simulink model "problem3_ccmodel"  (R2020a)
settings: Solver=VariableStepAuto  StartTime=0.0  StopTime=10.0  RelTol=1e-3
model workspace (MAT data in the model file):
  b = 50
  kd = 50
  ki = 300
  kp = 350
  m = 1000
  u = 500
settings Model: DataDictionary=poblem3_ccmodel.sldd  Creator=HP  LastModifiedBy=HP

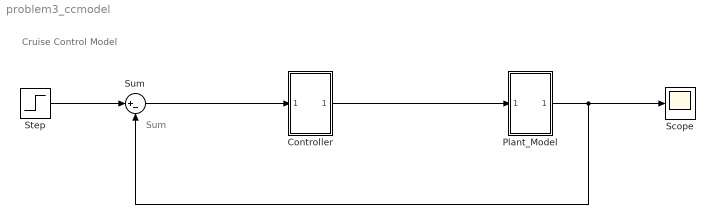
== system problem3_ccmodel ==
  note: Cruise Control Model
  note: Sum
  Controller : Subsystem  TreatAsAtomicUnit=on
  Plant_Model : Subsystem
  Scope : Scope
  Step : Step  Time=0  After=u  SampleTime=0
  Sum : Sum  Inputs=|+-
  wires:
  Step/1 -> Sum/1
  Plant_Model/1(Out1) -> Scope/1, Sum/2
  Sum/1 -> Controller/1(In1)
  Controller/1(Out1) -> Plant_Model/1(In1)

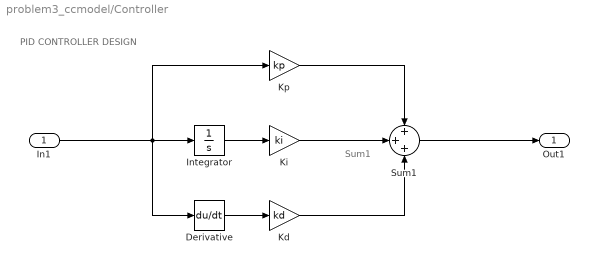
== system problem3_ccmodel/Controller ==
  note: PID CONTROLLER DESIGN
  note: Sum1
  In1 : Inport
  Derivative : Derivative
  Integrator : Integrator
  Kd : Gain  Gain=kd
  Ki : Gain  Gain=ki
  Kp : Gain  Gain=kp
  Sum1 : Sum  Inputs=+++
  Out1 : Outport
  wires:
  Ki/1 -> Sum1/2
  Derivative/1 -> Kd/1
  Kd/1 -> Sum1/3
  Integrator/1 -> Ki/1
  Sum1/1 -> Out1/1
  In1/1 -> Derivative/1, Integrator/1, Kp/1
  Kp/1 -> Sum1/1

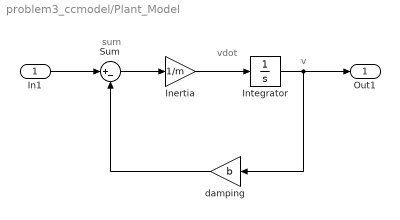
== system problem3_ccmodel/Plant_Model ==
  note: sum
  note: vdot
  note: v
  In1 : Inport
  Inertia : Gain  Gain=1/m
  Integrator : Integrator
  Sum : Sum  Inputs=|+-
  damping : Gain  Gain=b
  Out1 : Outport
  wires:
  Integrator/1 -> Out1/1, damping/1
  Sum/1 -> Inertia/1
  In1/1 -> Sum/1
  Inertia/1 -> Integrator/1
  damping/1 -> Sum/2
